simulink model "simulation"  (R2023b)
settings: Solver=VariableStepAuto  StartTime=0.0  StopTime=8  RelTol=1e-3
undefined symbols (not defined in the file or in its folder): Ki, Kp, pi_ctrl_tf_z_ba_neg, pi_ctrl_tf_z_fa_neg, pi_ctrl_tf_z_in_neg, pi_ctrl_tf_z_pzm_neg, pi_ctrl_tf_z_tus_neg, pi_ctrl_tf_z_zoh_neg
libraries: slpidlib x1
settings Model: Creator=camil  LastModifiedBy=camil

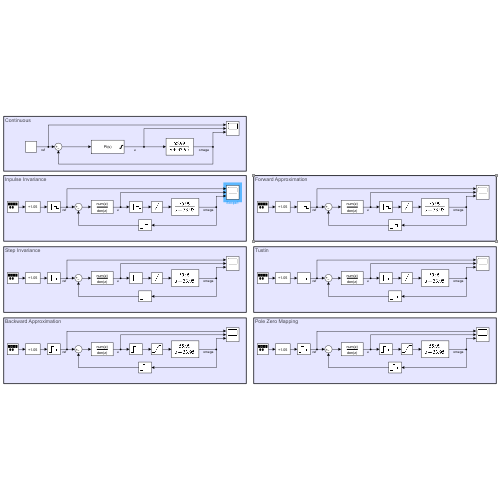
[thumbnail: Simulink's stored preview of the top-level diagram]
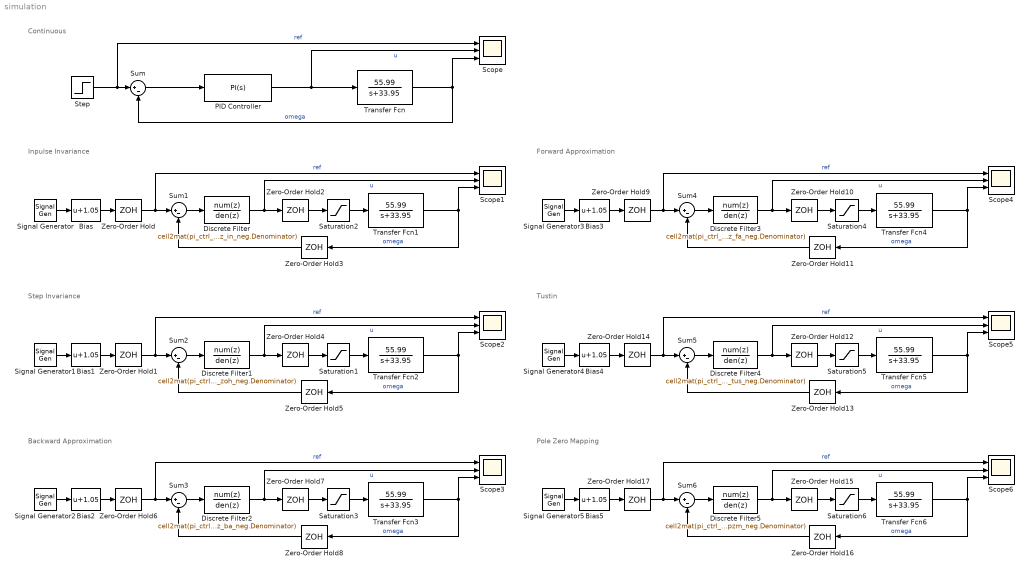
== system simulation ==
  note: Continuous
  note: Inpulse Invariance
  note: Step Invariance
  note: Backward Approximation
  note: Forward Approximation
  note: Tustin
  note: Pole Zero Mapping
  Bias{,1..5} (6 alike) : Bias  Bias=1.05  SaturateOnIntegerOverflow=off
  Discrete Filter : DiscreteFilter  Numerator=cell2mat(pi_ctrl_tf_z_in_neg.Numerator)  Denominator=cell2mat(pi_ctrl_tf_z_in_neg.Denominator)
  Discrete Filter1 : DiscreteFilter  Numerator=cell2mat(pi_ctrl_tf_z_zoh_neg.Numerator)  Denominator=cell2mat(pi_ctrl_tf_z_zoh_neg.Denominator)
  Discrete Filter2 : DiscreteFilter  Numerator=cell2mat(pi_ctrl_tf_z_ba_neg.Numerator)  Denominator=cell2mat(pi_ctrl_tf_z_ba_neg.Denominator)
  Discrete Filter3 : DiscreteFilter  Numerator=cell2mat(pi_ctrl_tf_z_fa_neg.Numerator)  Denominator=cell2mat(pi_ctrl_tf_z_fa_neg.Denominator)
  Discrete Filter4 : DiscreteFilter  Numerator=cell2mat(pi_ctrl_tf_z_tus_neg.Numerator)  Denominator=cell2mat(pi_ctrl_tf_z_tus_neg.Denominator)
  Discrete Filter5 : DiscreteFilter  Numerator=cell2mat(pi_ctrl_tf_z_pzm_neg.Numerator)  Denominator=cell2mat(pi_ctrl_tf_z_pzm_neg.Denominator)
  PID Controller : slpidlib/PID Controller  Controller=PI  Form=Parallel  TimeDomain=Continuous-time  UseExternalTs=off  SampleTime=-1  IntegratorMethod=Forward Euler  FilterMethod=Forward Euler  ControllerParametersSource=internal  P=Kp  I=Ki  UseKiTs=off  D=0  N=100  UseFilter=on  TunerSelectOption=Transfer Function Based (PID Tuner App)  InitialConditionSource=internal  InitialConditionForIntegrator=0  InitialConditionForFilter=0  DifferentiatorICPrevScaledInput=0  ExternalReset=none  TrackingMode=off  Kt=1  LimitOutput=on  SatLimitsSource=internal  UpperSaturationLimit=1  LowerSaturationLimit=-1  LinearizeAsGain=on  AntiWindupMode=none  Kb=1  LimitIntegrator=off  UpperIntegratorSaturationLimit=1  LowerIntegratorSaturationLimit=-inf  POutMin=[]  POutMax=[]  IOutMin=[]  IOutMax=[]  DOutMin=[]  DOutMax=[]  NOutMin=[]  NOutMax=[]  SumOutMin=[]  SumOutMax=[]  SaturationOutMin=[]  SaturationOutMax=[]  PParamMin=[]  PParamMax=[]  IParamMin=[]  IParamMax=[]  DParamMin=[]  DParamMax=[]  NParamMin=[]  NParamMax=[]  KbParamMin=[]  KbParamMax=[]  KtParamMin=[]  KtParamMax=[]  KbOutMin=[]  KbOutMax=[]  KtOutMin=[]  KtOutMax=[]  IntegratorOutMin=[]  IntegratorOutMax=[]  FilterOutMin=[]  FilterOutMax=[]  SumI1OutMin=[]  SumI1OutMax=[]  SumI2OutMin=[]  SumI2OutMax=[]  SumI3OutMin=[]  SumI3OutMax=[]  SumI4OutMin=[]  SumI4OutMax=[]  SumDOutMin=[]  SumDOutMax=[]  DifferentiatorOutMin=[]  DifferentiatorOutMax=[]  FilterDiffOutCoefMin=[]  FilterDiffOutCoefMax=[]  ReciprocalOutMin=[]  ReciprocalOutMax=[]  SumDenOutMin=[]  SumDenOutMax=[]  SumNumOutMin=[]  SumNumOutMax=[]  DivideOutMin=[]  DivideOutMax=[]  UdiffTsProdOutMin=[]  UdiffTsProdOutMax=[]  NTsProdOutMin=[]  NTsProdOutMax=[]  UintegralTsProdOutMin=[]  UintegralTsProdOutMax=[]  UngainTsProdOutMin=[]  UngainTsProdOutMax=[]  ClampingZeroOutDataTypeStr=Inherit: Inherit via back propagation  ClampingZeroOutMin=[]  ClampingZeroOutMax=[]  FilterDenConstantOutDataTypeStr=Inherit: Inherit via back propagation  FilterDenConstantOutMin=[]  FilterDenConstantOutMax=[]  PCopyOutDataTypeStr=Inherit: Inherit via back propagation  PCopyOutMin=[]  PCopyOutMax=[]  NCopyOutDataTypeStr=Inherit: Inherit via back propagation  NCopyOutMin=[]  NCopyOutMax=[]  IntegratorContinuousStateAttributes=''  IntegratorStateMustResolveToSignalObject=off  IntegratorRTWStateStorageClass=Auto  FilterContinuousStateAttributes=''  FilterStateMustResolveToSignalObject=off  FilterRTWStateStorageClass=Auto  ParallelPVariant=InternalParameters  IdealPVariant=Disabled  IVariant=InternalParameters  DVariant=Disabled  IntegratorVariant=Continuous  SatVariant=Enabled  AWVariant=Passthrough  PCopyVariant=Disabled  TRVariant=Disabled  FdbkBlocksVariant=Forward  IdealPFdbkVariant=Disabled  SatFdbkVariant=Disabled  DerivativeFilterVariant=Disabled  NVariant=Disabled  NCopyVariant=Disabled_SignalSpec  FilterICVariant=Disabled  IntegratorICVariant=InternalICs  ExternalResetVariant=Disabled  TRSumVariant=Passthrough  SumFdbkVariant=Disabled  SumVariant=Sum_PI  TsampFilterVariant=InternalTs  TsampNgainVariant=Passthrough  TsampIntegralVariant=Disabled_SignalSpec  ExternalSaturationOutDataTypeStr=Inherit: Same as second input
  Saturation{1..6} (6 alike) : Saturate  UpperLimit=1  LowerLimit=-1
  Scope{,1..6} (7 alike) : Scope  NumInputPorts=3
  Signal Generator{,1..5} (6 alike) : SignalGenerator  WaveForm=square  Amplitude=0.35  Frequency=0.25
  Step : Step  SampleTime=0.005
  Sum{,1..6} (7 alike) : Sum  Inputs=|+-
  Transfer Fcn{,1..6} (7 alike) : TransferFcn  Numerator=[55.99]  Denominator=[1 33.95]
  Zero-Order Hold{,1,6,9,14,17} (6 alike) : ZeroOrderHold  SampleTime=-1
  Zero-Order Hold{2..5,7..8,10..13,15..16} (12 alike) : ZeroOrderHold  SampleTime=0.005
  wires:
  Sum/1 -> PID Controller/1
  Step/1 -> Scope/1, Sum/1  "ref"
  Transfer Fcn/1 -> Scope/3, Sum/2  "omega"
  PID Controller/1 -> Scope/2, Transfer Fcn/1  "u"
  Zero-Order Hold3/1 -> Sum1/2
  Transfer Fcn1/1 -> Scope1/3, Zero-Order Hold3/1  "omega"
  Zero-Order Hold2/1 -> Saturation2/1
  Sum1/1 -> Discrete Filter/1
  Zero-Order Hold/1 -> Scope1/1, Sum1/1  "ref"
  Saturation2/1 -> Transfer Fcn1/1
  Discrete Filter/1 -> Scope1/2, Zero-Order Hold2/1  "u"
  Signal Generator/1 -> Bias/1
  Bias/1 -> Zero-Order Hold/1
  Bias1/1 -> Zero-Order Hold1/1
  Zero-Order Hold1/1 -> Scope2/1, Sum2/1  "ref"
  Zero-Order Hold5/1 -> Sum2/2
  Transfer Fcn2/1 -> Scope2/3, Zero-Order Hold5/1  "omega"
  Zero-Order Hold4/1 -> Saturation1/1
  Signal Generator1/1 -> Bias1/1
  Sum2/1 -> Discrete Filter1/1
  Discrete Filter1/1 -> Scope2/2, Zero-Order Hold4/1  "u"
  Saturation1/1 -> Transfer Fcn2/1
  Saturation3/1 -> Transfer Fcn3/1
  Sum3/1 -> Discrete Filter2/1
  Signal Generator2/1 -> Bias2/1
  Zero-Order Hold7/1 -> Saturation3/1
  Discrete Filter2/1 -> Scope3/2, Zero-Order Hold7/1  "u"
  Transfer Fcn3/1 -> Scope3/3, Zero-Order Hold8/1  "omega"
  Zero-Order Hold8/1 -> Sum3/2
  Zero-Order Hold6/1 -> Scope3/1, Sum3/1  "ref"
  Bias2/1 -> Zero-Order Hold6/1
  Bias3/1 -> Zero-Order Hold9/1
  Zero-Order Hold9/1 -> Scope4/1, Sum4/1  "ref"
  Saturation4/1 -> Transfer Fcn4/1
  Zero-Order Hold10/1 -> Saturation4/1
  Sum4/1 -> Discrete Filter3/1
  Zero-Order Hold11/1 -> Sum4/2
  Discrete Filter3/1 -> Scope4/2, Zero-Order Hold10/1  "u"
  Transfer Fcn4/1 -> Scope4/3, Zero-Order Hold11/1  "omega"
  Signal Generator3/1 -> Bias3/1
  Discrete Filter4/1 -> Scope5/2, Zero-Order Hold12/1  "u"
  Sum5/1 -> Discrete Filter4/1
  Transfer Fcn5/1 -> Scope5/3, Zero-Order Hold13/1  "omega"
  Signal Generator4/1 -> Bias4/1
  Saturation5/1 -> Transfer Fcn5/1
  Bias4/1 -> Zero-Order Hold14/1
  Zero-Order Hold14/1 -> Scope5/1, Sum5/1  "ref"
  Zero-Order Hold12/1 -> Saturation5/1
  Zero-Order Hold13/1 -> Sum5/2
  Zero-Order Hold17/1 -> Scope6/1, Sum6/1  "ref"
  Zero-Order Hold16/1 -> Sum6/2
  Zero-Order Hold15/1 -> Saturation6/1
  Sum6/1 -> Discrete Filter5/1
  Bias5/1 -> Zero-Order Hold17/1
  Saturation6/1 -> Transfer Fcn6/1
  Signal Generator5/1 -> Bias5/1
  Transfer Fcn6/1 -> Scope6/3, Zero-Order Hold16/1  "omega"
  Discrete Filter5/1 -> Scope6/2, Zero-Order Hold15/1  "u"
